simulink model "orbit"  (R2019b)
settings: Solver=ode45  StartTime=0.0  StopTime=simTime  RelTol=1e-4
values from neighbouring files (symbols this model uses):
  a = zeros(2,1)    [init.m]
  b = zeros(2,1)    [init.m]
  c = zeros(2,1)    [init.m]
  disturbance = 1    [init.m]
  Gsc = 1360.8    [init.m]
  h = zeros(2,1)    [init.m]
  k = 0.1    [init.m]
  L2 = 1.1556    [init.m]
  mu = 0.012149    [init.m]
  Omega = 1.8636    [init.m]
  Omega_z = Omega    (= 1.8636)    [init.m]
  phi = 0    [init.m]
  ref_select = 1    [init.m]
  sped = 300000    [init.m]
  srp = 1    [init.m]
  u0 = [0;0;0]    [init.m]
  x0 = [L2;0;0;0;0;0]    [init.m]
  zeta = 0.9252    [init.m]
settings Model: Creator=mohd-  LastModifiedBy=mohd-

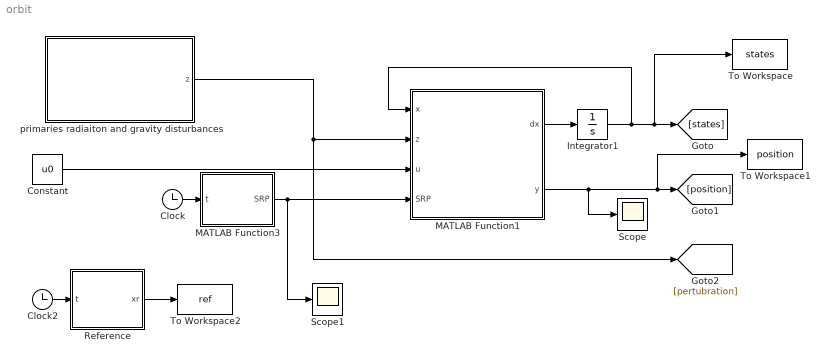
== system orbit ==
  Clock : Clock
  Clock2 : Clock
  Constant : Constant  Value=u0
  Integrator1 : Integrator  InitialCondition=x0
  MATLAB Function1 : MATLAB Function  TreatAsAtomicUnit=on
  MATLAB Function3 : MATLAB Function  TreatAsAtomicUnit=on
  Reference : MATLAB Function  TreatAsAtomicUnit=on
  Scope : Scope
  Scope1 : Scope
  To Workspace : ToWorkspace  VariableName=states  SampleTime=10^-3
      settings: Save2DSignal=2-D array (concatenate along first dimension)
  To Workspace1 : ToWorkspace  VariableName=position  SampleTime=10^-3
      settings: Save2DSignal=2-D array (concatenate along first dimension)
  To Workspace2 : ToWorkspace  VariableName=ref  SampleTime=10^-3
      settings: Save2DSignal=2-D array (concatenate along first dimension)
  primaries radiaiton and gravity disturbances : Subsystem
  wires:
  primaries radiaiton and gravity disturbances/1(z) -> [pertubration], MATLAB Function1/2(z)
  Constant/1 -> MATLAB Function1/3(u)
  Clock/1 -> MATLAB Function3/1(t)
  MATLAB Function1/2(y) -> To Workspace1/1, [position], Scope/1
  Integrator1/1 -> To Workspace/1, [states], MATLAB Function1/1(x)
  MATLAB Function1/1(dx) -> Integrator1/1
  MATLAB Function3/1(SRP) -> Scope1/1, MATLAB Function1/4(SRP)
  Clock2/1 -> Reference/1(t)
  Reference/1(xr) -> To Workspace2/1

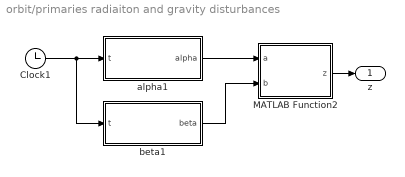
== system orbit/primaries radiaiton and gravity disturbances ==
  Clock1 : Clock
  MATLAB Function2 : MATLAB Function  TreatAsAtomicUnit=on
  alpha1 : MATLAB Function  TreatAsAtomicUnit=on
  beta1 : MATLAB Function  TreatAsAtomicUnit=on
  z : Outport
  wires:
  Clock1/1 -> beta1/1(t), alpha1/1(t)
  beta1/1(beta) -> MATLAB Function2/2(b)
  alpha1/1(alpha) -> MATLAB Function2/1(a)
  MATLAB Function2/1(z) -> z/1

== matlab function orbit/MATLAB Function1 ==
  data: x input; z input; dx output; u input; y output; mu parameter; SRP input
function [dx, y] = Satellite(x,z, u, mu, SRP)

x1 = x(1:3);
x2 = x(4:6);

M = [-1 0 0;
    0 -1 0;
    0 0 0];

N = [0 -1 0;
    1 0 0;
    0 0 0];

d1r = [-mu - z(4)/(1-mu);0;0];
d2r = [1-mu + z(4)/mu;0;0];

ed1 = x1 - d1r;
absed1 = sqrt(ed1(1)^2+ed1(2)^2+ed1(3)^2);
ed2 = x1 - d2r;
absed2 = sqrt(ed2(1)^2+ed2(2)^2+ed2(3)^2);

f1 = x2;
f2 = -M*x1 - 2*N*x2 - (2*M*x1 + 2*N*x2)*z(1) ...
           - M*x1*z(2) - N*x1*z(3) - ed1*(1 - mu)/absed1^3 ...
           - ed2*mu/absed2^3;
F = [f1; f2 + SRP];
G = [zeros(3); eye(3)];


dx = F + G*u;
y  = x1;

== matlab function orbit/Reference ==
  data: t input; xr output; k parameter; c parameter; Omega parameter; Omega_z parameter; L2 parameter; h parameter; ref_select parameter; phi parameter
function xr = refer(t,k,c,Omega,Omega_z,L2,h,ref_select,phi)
%#codegen

Seq = [L2;0;0;0;0;0];
e = exp(1);

ho1 = [(-k*(1-c(1)+Omega^2)/(2*Omega))*cos(Omega*t);
       k*sin(Omega*t);
       k*cos(Omega_z*t)];
   
diffho1 = [(k*(1-c(1)+Omega^2)/2)*sin(Omega*t);
           Omega*k*cos(Omega*t);
           -Omega_z*k*sin(Omega_z*t)];
       
ho2 = ho1 + [e*h(1)*cos(t+phi);
             e*h(2)*sin(t+phi);
             0];
         
diffho2 = diffho1 + [-e*h(1)*sin(t+phi);
                    e*h(2)*cos(t+phi);
                    0];
xr = Seq;
%xr = zeros(6,1);
if ref_select == 1
    xr = xr + [ho1;diffho1];
else
    xr = xr + [ho2;diffho2];
end

== matlab function orbit/MATLAB Function3 ==
  data: SRP output; srp parameter; Gsc parameter; sped parameter; zeta parameter; t input
function SRP = fcn(srp, Gsc, sped, zeta,t)

if srp == 1
    SRP = [(Gsc/sped)*(cos(zeta*t))^2;(Gsc/sped)*(sin(zeta*t))^2;0];
else
    SRP = [0;0;0];
end

== matlab function orbit/primaries radiaiton and gravity disturbances/MATLAB Function2 ==
  data: a input; z output; b input; mu parameter; disturbance parameter
function z = z(a,b,mu, disturbance)
%#codegen
if disturbance == 1
    z = [b;mu*(1-mu)*a];
else
    z = zeros(4,1);
end

== matlab function orbit/primaries radiaiton and gravity disturbances/alpha1 ==
  data: t input; alpha output; a parameter; phi parameter; e parameter
function alpha = a(t,a,phi,e)
%#codegen

a1 = a(1)*e*cos(t+phi);
alpha = a1;

== matlab function orbit/primaries radiaiton and gravity disturbances/beta1 ==
  data: t input; beta output; b parameter; phi parameter; e parameter
function beta = b(t,b,phi,e)
%#codegen
b1 = b(1)*e*cos(t+phi);
bd = -b(1)*e*sin(t+phi);
beta = [b1;0;bd];
